simulink model "reshape_test"  (Simulink 9.0)
settings: Solver=FixedStepAuto  StartTime=0.0  StopTime=10.0  FixedStep=0.1  RelTol=1e-3  EnableMultiTasking=on
settings Model: SuppressorTable=22 serialization::archive 11 0 6 0 0 0 0 0  Creator=arnaud  LastModifiedBy=hbourbou
settings DataIOCC: LimitDataPoints=on  SaveFormat=Structure  SignalLoggingSaveFormat=ModelDataLogs
settings OptimizationCC: ExpressionDepthLimit=2147483647
settings DebuggingCC: SolverPrmCheckMsg=warning  FcnCallInpInsideContextMsg=warning  StateNameClashWarn=warning
settings GRTTargetCC: GeneratePreprocessorConditionals=Disable all  CombineOutputUpdateFcns=off  GRTInterface=on
settings ConfigComp: CovSFcnEnable=off

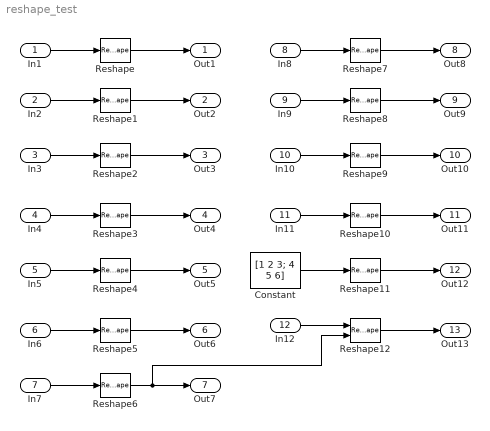
== system reshape_test ==
  In1 : Inport  OutDataTypeStr=double  PortDimensions=1
  In2 : Inport  Port=2  PortDimensions=5
  In3 : Inport  Port=3  OutDataTypeStr=boolean  PortDimensions=[2 3]
  In4 : Inport  Port=4  PortDimensions=5
  In5 : Inport  Port=5  OutDataTypeStr=boolean  PortDimensions=[2 3]
  In6 : Inport  Port=6  PortDimensions=5
  In7 : Inport  Port=7  OutDataTypeStr=boolean  PortDimensions=[2 3]
  In8 : Inport  Port=8  PortDimensions=5
  In9 : Inport  Port=9  OutDataTypeStr=boolean  PortDimensions=[2 3]
  In10 : Inport  Port=10  OutDataTypeStr=boolean  PortDimensions=[2 3]
  In11 : Inport  Port=11  OutDataTypeStr=boolean  PortDimensions=[2 3]
  In12 : Inport  Port=12  OutDataTypeStr=boolean  PortDimensions=[2 3]
  Constant : Constant  Value=[1 2 3; 4 5 6]
  Reshape : Reshape
  Reshape1 : Reshape
  Reshape10 : Reshape  OutputDimensionality=Customize  OutputDimensions=[6,1]
  Reshape11 : Reshape  OutputDimensionality=Customize  OutputDimensions=[3,2]
  Reshape12 : Reshape  OutputDimensionality=Derive from reference input port  OutputDimensions=[6,1]
  Reshape2 : Reshape
  Reshape3 : Reshape  OutputDimensionality=Column vector (2-D)
  Reshape4 : Reshape  OutputDimensionality=Column vector (2-D)
  Reshape5 : Reshape  OutputDimensionality=Row vector (2-D)
  Reshape6 : Reshape  OutputDimensionality=Row vector (2-D)
  Reshape7 : Reshape  OutputDimensionality=Customize  OutputDimensions=[5]
  Reshape8 : Reshape  OutputDimensionality=Customize  OutputDimensions=[1,6]
  Reshape9 : Reshape  OutputDimensionality=Customize  OutputDimensions=[6]
  Out1 : Outport
  Out2 : Outport  Port=2
  Out3 : Outport  Port=3
  Out4 : Outport  Port=4
  Out5 : Outport  Port=5
  Out6 : Outport  Port=6
  Out7 : Outport  Port=7
  Out8 : Outport  Port=8
  Out9 : Outport  Port=9
  Out10 : Outport  Port=10
  Out11 : Outport  Port=11
  Out12 : Outport  Port=12
  Out13 : Outport  Port=13
  wires:
  Reshape/1 -> Out1/1
  In1/1 -> Reshape/1
  In2/1 -> Reshape1/1
  Reshape1/1 -> Out2/1
  In3/1 -> Reshape2/1
  Reshape2/1 -> Out3/1
  In4/1 -> Reshape3/1
  Reshape3/1 -> Out4/1
  In5/1 -> Reshape4/1
  Reshape4/1 -> Out5/1
  In6/1 -> Reshape5/1
  Reshape5/1 -> Out6/1
  In7/1 -> Reshape6/1
  Reshape6/1 -> Reshape12/2, Out7/1
  In8/1 -> Reshape7/1
  Reshape7/1 -> Out8/1
  In9/1 -> Reshape8/1
  Reshape8/1 -> Out9/1
  In10/1 -> Reshape9/1
  Reshape9/1 -> Out10/1
  In11/1 -> Reshape10/1
  Reshape10/1 -> Out11/1
  Reshape11/1 -> Out12/1
  Constant/1 -> Reshape11/1
  In12/1 -> Reshape12/1
  Reshape12/1 -> Out13/1
